simulink model "car_model_friction"  (Simulink 7.5)
settings: Solver=ode3  StartTime=0.0  StopTime=20  FixedStep=0.01  RelTol=1e-3
undefined symbols (not defined in the file or in its folder): X0
settings Model: Creator=oktay  LastModifiedBy=oktay

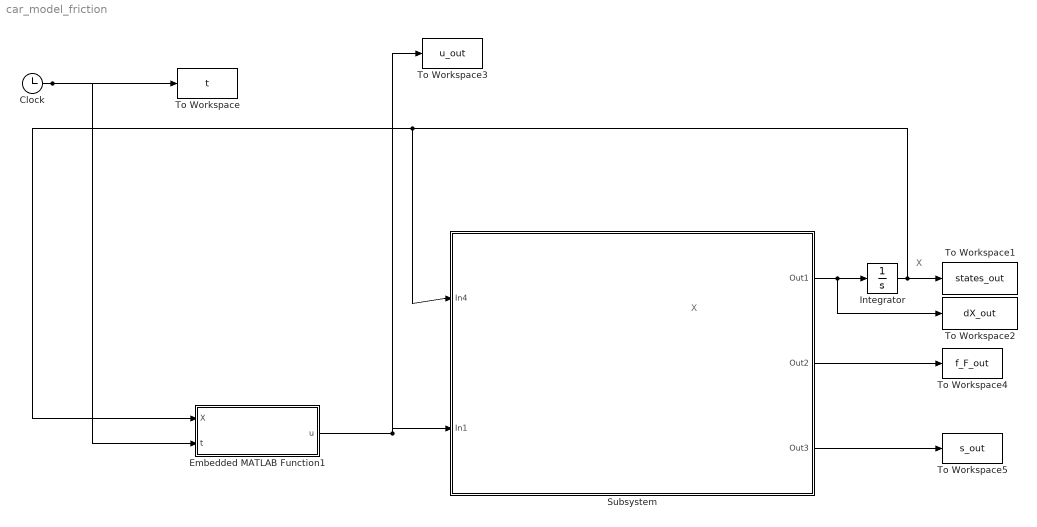
== system car_model_friction ==
  note: X
  note: X
  Clock : Clock
      settings: Decimation=10
  Embedded MATLAB Function1 : Stateflow chart  TreatAsAtomicUnit=on
  Integrator : Integrator  InitialCondition=X0
  Subsystem : Subsystem
      mask Display: image(imread('car_logo.png'))
  To Workspace : ToWorkspace  VariableName=t  SampleTime=-1  SaveFormat=Array
  To Workspace1 : ToWorkspace  VariableName=states_out  SampleTime=-1  SaveFormat=Array
  To Workspace2 : ToWorkspace  VariableName=dX_out  SampleTime=-1  SaveFormat=Array
  To Workspace3 : ToWorkspace  VariableName=u_out  SampleTime=-1  SaveFormat=Array
  To Workspace4 : ToWorkspace  VariableName=f_F_out  SampleTime=-1  SaveFormat=Array
  To Workspace5 : ToWorkspace  VariableName=s_out  SampleTime=-1  SaveFormat=Array
  wires:
  Subsystem/1(Out1) -> Integrator/1, To Workspace2/1
  Embedded MATLAB Function1/1(u) -> Subsystem/2(In1), To Workspace3/1
  Integrator/1 -> To Workspace1/1, Embedded MATLAB Function1/1(X), Subsystem/1(In4)
  Clock/1 -> To Workspace/1, Embedded MATLAB Function1/2(t)
  Subsystem/2(Out2) -> To Workspace4/1
  Subsystem/3(Out3) -> To Workspace5/1

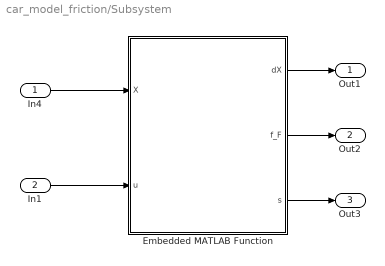
== system car_model_friction/Subsystem ==
  In4 : Inport
  In1 : Inport  Port=2
  Embedded MATLAB Function : Stateflow chart  TreatAsAtomicUnit=on
  Out1 : Outport
  Out2 : Outport  Port=2
  Out3 : Outport  Port=3
  wires:
  In1/1 -> Embedded MATLAB Function/2(u)
  Embedded MATLAB Function/1(dX) -> Out1/1
  In4/1 -> Embedded MATLAB Function/1(X)
  Embedded MATLAB Function/2(f_F) -> Out2/1
  Embedded MATLAB Function/3(s) -> Out3/1

== matlab function Embedded MATLAB Function1 ==
  data: u output double; X input double; t input double
function u = controller(X,t)
%#eml
global CONSTANTS

f_Fx = -2000;
f_Rx = -2000;



delta = 45*pi/180*sin(2*pi/10*t);
u = [f_Fx; f_Rx; delta];

== matlab function Subsystem/Embedded MATLAB Function ==
  data: X input double; u input double; dX output double; f_F output double; s output double
function [dX, f_F, s ] = car_dynamics(X, u )


    g = 9.82;
    m = 1450;
    Iz = 2740;
    l_F = 1.1;
    l_R = 1.6;
    B = 7;
    C = 1.4;
    mu = 0.5;
    f_Fz = m*g*l_R*(l_F + l_R);
    f_Rz = m*g*l_F*(l_F + l_R);

    kmh2ms = 10/36;
    ms2kmh = 36/10;
    deg2rad = pi/180;
    rad2deg = 180/pi;

    % Minimum and maximum values of the controls

    f_Fx_min = -mu*f_Fz + 2000;
    f_Fx_max = 0; 

    f_Rx_min = -mu*f_Rz + 2000;
    f_Rx_max = mu*f_Rz - 2000;

    Vx  = X(1);
    Vy  = X(2);
    r   = X(3);
    psi = X(4);
    xi  = X(5);
    yi  = X(6);


    f_Fx  = u(1);
    f_Rx  = u(2);
    delta = u(3);

    mu = mu;
    
    Vxw = cos(delta).*Vx + sin(delta).*Vy;
    Vyw = -sin(delta).*Vx + cos(delta).*Vy;

    if ( f_Fx >= 0)
        f_Fx = 0;
    elseif (f_Fx <= -mu*f_Fz)
        f_Fx = -mu*f_Fz;
    end

    f_Fx = f_Fx*sign(Vxw);

    if ( f_Rx >= mu*f_Rz)
        f_Rx =  mu*f_Rz;
    elseif (f_Rx <= -mu*f_Rz)
        f_Rx = -mu*f_Rz;
    end

    if (f_Rx < 0)   % braking request
        f_Rx = sign(Vx)*f_Rx;
    end

    if ( delta >= 45*pi/180)
        delta = 45*pi/180;
    elseif (delta <= -45*pi/180)
        delta = -45*pi/180;
    end

    %Auxiliar variables
    V = sqrt(Vx.^2+Vy.^2);
    beta = atan2(Vy,Vx);

    f_Fy_max = sqrt( (mu*f_Fz).^2 - f_Fx.^2 );
    s_Fy = (V.*sin(beta-delta)+r*l_F.*cos(delta))./(V.*cos(beta-delta)+r*l_F.*sin(delta));

    if (V < 0.8)
        s_Fy = 0;
    end

    f_Fy = -f_Fy_max.*sin(C*atan(B*s_Fy));


    f_Ry_max = sqrt( (mu*f_Rz).^2 - f_Rx.^2 );
    s_Ry =(V.*sin(beta)-r*l_R)./(V.*cos(beta));

    if (V < 0.8)
        s_Ry = 0;
    end

    f_Ry = -f_Ry_max.*sin(C*atan(B*s_Ry));


    dVx = 1/m.*(f_Fx.*cos(delta) - f_Fy.*sin(delta) + f_Rx) + Vy.*r;
    dVy = 1/m.*(f_Fx.*sin(delta) + f_Fy.*cos(delta) + f_Ry) - Vx.*r;
    dr = 1/Iz.*((f_Fy.*cos(delta) + f_Fx.*sin(delta)).*l_F - f_Ry.*l_R);
    dpsi = r;
    dxi = cos(psi).*Vx - sin(psi).*Vy;
    dyi = sin(psi).*Vx + cos(psi).*Vy;

    dX = [dVx dVy dr dpsi dxi dyi]';
    
    s = [s_Fy s_Ry]';
    
    f_F = [f_Fy f_Ry]';
    
end
